simulink model "My_Model"  (R2022a)
settings: Solver=VariableStepAuto  StartTime=0.0  StopTime=10.0  RelTol=1e-3
libraries: neural x1294, spsSeriesRLCBranchLib x16, spsDiodeLib x14, spsMosfetLib x9, spsVoltageMeasurementLib x9, powerlib_extras x8, spsThreePhaseVIMeasurementLib x7, spsCurrentMeasurementLib x4, spsPVArrayLib x4, spsPWMGeneratorDCDCLib x4, spsTHDLib x4, spsThreePhaseParallelRLCBranchLib x3
(part 35 of 41)

== system My_Model/VSC Control/Current Regulator/7 layer network/Layer 3/LW{3,1} ==
  "ad{3,1}" : Inport  PortDimensions=5
      mask Display: e = 0.06;c1 = [120 230 180]/255;c2 = ([120 230 180]+0)/(256+128);c3 = ([120 230 180]+128)/(256+128);patch([0 1 1 0],[0 0 1 1],c1);patch([0 1 1 1-e 1-e 0+e],[0 0 1 1-e 0+e 0+e],c2);patch([0 0 1 1-e 0+e 0+e],[0 1 1 1-e 1-e 0+e],c3);plot([0 1 1 0 0],[0 0 1 1 0]);
  "IW{3,1}(1,:)'" : Constant  Value=[-1.8648429690334877850688144462765194475650787353515625;1.64641616981970440036775471526198089122772216796875;1.3574904436003685237466243052040226757526397705078125;0.1951467267628609059126887359525426290929317474365234375;0.67017177325838772627975004070322029292583465576171875]
      mask Display: e = 0.06;c1 = [120 150 230]/255;c2 = ([120 150 230]+0)/383;c3 = ([120 150 230]+128)/383;patch([0 1 1 0],[0 0 1 1],c1);patch([0 1 1 1-e 1-e 0+e],[0 0 1 1-e 0+e 0+e],c2);patch([0 0 1 1-e 0+e 0+e],[0 1 1 1-e 1-e 0+e],c3);plot([0 1 1 0 0],[0 0 1 1 0]);disp('weights');
  "IW{3,1}(10,:)'" : Constant  Value=[1.730384337449465181890673193265683948993682861328125;-1.493153814263745715607001329772174358367919921875;-2.530359722244460041196134625351987779140472412109375;-2.40776132219388561139794546761550009250640869140625;0.50114335757025896267435882691643200814723968505859375]
      mask Display: e = 0.06;c1 = [120 150 230]/255;c2 = ([120 150 230]+0)/383;c3 = ([120 150 230]+128)/383;patch([0 1 1 0],[0 0 1 1],c1);patch([0 1 1 1-e 1-e 0+e],[0 0 1 1-e 0+e 0+e],c2);patch([0 0 1 1-e 0+e 0+e],[0 1 1 1-e 1-e 0+e],c3);plot([0 1 1 0 0],[0 0 1 1 0]);disp('weights');
  "IW{3,1}(11,:)'" : Constant  Value=[-0.372842919851827547805811491343774832785129547119140625;-0.5046690348264208925144203021773137152194976806640625;-1.515886409077602525741212957655079662799835205078125;2.468679428778111084596957880421541631221771240234375;-1.7226432394641111311983650011825375258922576904296875]
      mask Display: e = 0.06;c1 = [120 150 230]/255;c2 = ([120 150 230]+0)/383;c3 = ([120 150 230]+128)/383;patch([0 1 1 0],[0 0 1 1],c1);patch([0 1 1 1-e 1-e 0+e],[0 0 1 1-e 0+e 0+e],c2);patch([0 0 1 1-e 0+e 0+e],[0 1 1 1-e 1-e 0+e],c3);plot([0 1 1 0 0],[0 0 1 1 0]);disp('weights');
  "IW{3,1}(12,:)'" : Constant  Value=[2.43443382104679617583542494685389101505279541015625;-2.69250576871099323028602157137356698513031005859375;-0.8594546905821596194385847411467693746089935302734375;1.642889282015585816765224080882035195827484130859375;-1.18668618700788908171261937241069972515106201171875]
      mask Display: e = 0.06;c1 = [120 150 230]/255;c2 = ([120 150 230]+0)/383;c3 = ([120 150 230]+128)/383;patch([0 1 1 0],[0 0 1 1],c1);patch([0 1 1 1-e 1-e 0+e],[0 0 1 1-e 0+e 0+e],c2);patch([0 0 1 1-e 0+e 0+e],[0 1 1 1-e 1-e 0+e],c3);plot([0 1 1 0 0],[0 0 1 1 0]);disp('weights');
  "IW{3,1}(13,:)'" : Constant  Value=[-1.866170167135730917351565949502401053905487060546875;2.372303607311231576915133700822480022907257080078125;1.88285380700856563862544135190546512603759765625;-0.057789596629258331572653872854061773978173732757568359375;-0.1485964355318751539680732776105287484824657440185546875]
      mask Display: e = 0.06;c1 = [120 150 230]/255;c2 = ([120 150 230]+0)/383;c3 = ([120 150 230]+128)/383;patch([0 1 1 0],[0 0 1 1],c1);patch([0 1 1 1-e 1-e 0+e],[0 0 1 1-e 0+e 0+e],c2);patch([0 0 1 1-e 0+e 0+e],[0 1 1 1-e 1-e 0+e],c3);plot([0 1 1 0 0],[0 0 1 1 0]);disp('weights');
  "IW{3,1}(14,:)'" : Constant  Value=[-1.22626251288648457915542167029343545436859130859375;2.309849211314865424782283298554830253124237060546875;-2.4839196222544988046365688205696642398834228515625;-0.35577383199778978006833085601101629436016082763671875;-1.38721598608713492239985498599708080291748046875]
      mask Display: e = 0.06;c1 = [120 150 230]/255;c2 = ([120 150 230]+0)/383;c3 = ([120 150 230]+128)/383;patch([0 1 1 0],[0 0 1 1],c1);patch([0 1 1 1-e 1-e 0+e],[0 0 1 1-e 0+e 0+e],c2);patch([0 0 1 1-e 0+e 0+e],[0 1 1 1-e 1-e 0+e],c3);plot([0 1 1 0 0],[0 0 1 1 0]);disp('weights');
  "IW{3,1}(15,:)'" : Constant  Value=[-2.172691293821853886214512385777197778224945068359375;-0.0555052400358548581049689119026879779994487762451171875;-2.796772108373029031014311840408481657505035400390625;-0.322606729897259025818812006036750972270965576171875;2.110627404777451143758071339107118546962738037109375]
      mask Display: e = 0.06;c1 = [120 150 230]/255;c2 = ([120 150 230]+0)/383;c3 = ([120 150 230]+128)/383;patch([0 1 1 0],[0 0 1 1],c1);patch([0 1 1 1-e 1-e 0+e],[0 0 1 1-e 0+e 0+e],c2);patch([0 0 1 1-e 0+e 0+e],[0 1 1 1-e 1-e 0+e],c3);plot([0 1 1 0 0],[0 0 1 1 0]);disp('weights');
  "IW{3,1}(16,:)'" : Constant  Value=[-1.8000723946908561146074134740047156810760498046875;-0.049744368180471336404746551806965726427733898162841796875;-1.6945002191867055696405941489501856267452239990234375;-0.93860331245166783720179637384717352688312530517578125;-1.5469042667476922137126393863582052290439605712890625]
      mask Display: e = 0.06;c1 = [120 150 230]/255;c2 = ([120 150 230]+0)/383;c3 = ([120 150 230]+128)/383;patch([0 1 1 0],[0 0 1 1],c1);patch([0 1 1 1-e 1-e 0+e],[0 0 1 1-e 0+e 0+e],c2);patch([0 0 1 1-e 0+e 0+e],[0 1 1 1-e 1-e 0+e],c3);plot([0 1 1 0 0],[0 0 1 1 0]);disp('weights');
  "IW{3,1}(17,:)'" : Constant  Value=[2.649656781046310971561297264997847378253936767578125;-1.128764384600953629700370584032498300075531005859375;0.99796670093458150763154890228179283440113067626953125;-0.014251502504089512413099072318800608627498149871826171875;-2.028262431616330463413078177836723625659942626953125]
      mask Display: e = 0.06;c1 = [120 150 230]/255;c2 = ([120 150 230]+0)/383;c3 = ([120 150 230]+128)/383;patch([0 1 1 0],[0 0 1 1],c1);patch([0 1 1 1-e 1-e 0+e],[0 0 1 1-e 0+e 0+e],c2);patch([0 0 1 1-e 0+e 0+e],[0 1 1 1-e 1-e 0+e],c3);plot([0 1 1 0 0],[0 0 1 1 0]);disp('weights');
  "IW{3,1}(18,:)'" : Constant  Value=[0.469414061379627545189663351266062818467617034912109375;2.49243645667582303104836682905443012714385986328125;1.427744966641751656055703278980217874050140380859375;0.1331815618988561322755259652694803662598133087158203125;-2.0229494597613353334963903762400150299072265625]
      mask Display: e = 0.06;c1 = [120 150 230]/255;c2 = ([120 150 230]+0)/383;c3 = ([120 150 230]+128)/383;patch([0 1 1 0],[0 0 1 1],c1);patch([0 1 1 1-e 1-e 0+e],[0 0 1 1-e 0+e 0+e],c2);patch([0 0 1 1-e 0+e 0+e],[0 1 1 1-e 1-e 0+e],c3);plot([0 1 1 0 0],[0 0 1 1 0]);disp('weights');
  "IW{3,1}(19,:)'" : Constant  Value=[0.281291509588638410921390686780796386301517486572265625;-0.73770186006364502073751054922468028962612152099609375;0.83145324988802282728528325606021098792552947998046875;1.7885333638585640958496014718548394739627838134765625;-1.539351153646769443383846009965054690837860107421875]
      mask Display: e = 0.06;c1 = [120 150 230]/255;c2 = ([120 150 230]+0)/383;c3 = ([120 150 230]+128)/383;patch([0 1 1 0],[0 0 1 1],c1);patch([0 1 1 1-e 1-e 0+e],[0 0 1 1-e 0+e 0+e],c2);patch([0 0 1 1-e 0+e 0+e],[0 1 1 1-e 1-e 0+e],c3);plot([0 1 1 0 0],[0 0 1 1 0]);disp('weights');
  "IW{3,1}(2,:)'" : Constant  Value=[2.647424845222875244843407926964573562145233154296875;0.706534071197615798354263461078517138957977294921875;-0.6292432117475985631216417459654621779918670654296875;-1.1688666566529841706056913608335889875888824462890625;-0.69896032812457409288953158466028980910778045654296875]
      mask Display: e = 0.06;c1 = [120 150 230]/255;c2 = ([120 150 230]+0)/383;c3 = ([120 150 230]+128)/383;patch([0 1 1 0],[0 0 1 1],c1);patch([0 1 1 1-e 1-e 0+e],[0 0 1 1-e 0+e 0+e],c2);patch([0 0 1 1-e 0+e 0+e],[0 1 1 1-e 1-e 0+e],c3);plot([0 1 1 0 0],[0 0 1 1 0]);disp('weights');
  "IW{3,1}(20,:)'" : Constant  Value=[-2.23870144087298594826052067219279706478118896484375;-2.4681369116425884158161352388560771942138671875;-0.327772930287947350525001866117236204445362091064453125;1.7867146454480125061792250562575645744800567626953125;-0.5014624623065147002165531375794671475887298583984375]
      mask Display: e = 0.06;c1 = [120 150 230]/255;c2 = ([120 150 230]+0)/383;c3 = ([120 150 230]+128)/383;patch([0 1 1 0],[0 0 1 1],c1);patch([0 1 1 1-e 1-e 0+e],[0 0 1 1-e 0+e 0+e],c2);patch([0 0 1 1-e 0+e 0+e],[0 1 1 1-e 1-e 0+e],c3);plot([0 1 1 0 0],[0 0 1 1 0]);disp('weights');
  "IW{3,1}(3,:)'" : Constant  Value=[-2.659172848885479112368557252921164035797119140625;-0.79211056958587333642896055607707239687442779541015625;-1.3825222862382287036808747870963998138904571533203125;1.425055984082430615700332054984755814075469970703125;1.8025932077864765812336145245353691279888153076171875]
      mask Display: e = 0.06;c1 = [120 150 230]/255;c2 = ([120 150 230]+0)/383;c3 = ([120 150 230]+128)/383;patch([0 1 1 0],[0 0 1 1],c1);patch([0 1 1 1-e 1-e 0+e],[0 0 1 1-e 0+e 0+e],c2);patch([0 0 1 1-e 0+e 0+e],[0 1 1 1-e 1-e 0+e],c3);plot([0 1 1 0 0],[0 0 1 1 0]);disp('weights');
  "IW{3,1}(4,:)'" : Constant  Value=[1.8265068772120660600677410911885090172290802001953125;0.08917576894467467429894469432838377542793750762939453125;-0.63678331617796046781876384557108394801616668701171875;-2.063555639273333408567623337148688733577728271484375;0.2208531191929975767695992772132740356028079986572265625]
      mask Display: e = 0.06;c1 = [120 150 230]/255;c2 = ([120 150 230]+0)/383;c3 = ([120 150 230]+128)/383;patch([0 1 1 0],[0 0 1 1],c1);patch([0 1 1 1-e 1-e 0+e],[0 0 1 1-e 0+e 0+e],c2);patch([0 0 1 1-e 0+e 0+e],[0 1 1 1-e 1-e 0+e],c3);plot([0 1 1 0 0],[0 0 1 1 0]);disp('weights');
  "IW{3,1}(5,:)'" : Constant  Value=[1.5732001173784180281245426158420741558074951171875;-0.43016677249347023970216241650632582604885101318359375;-2.027900356396983294615665727178566157817840576171875;1.0006433005602011210299906451837159693241119384765625;-0.72263860216961794957768461244995705783367156982421875]
      mask Display: e = 0.06;c1 = [120 150 230]/255;c2 = ([120 150 230]+0)/383;c3 = ([120 150 230]+128)/383;patch([0 1 1 0],[0 0 1 1],c1);patch([0 1 1 1-e 1-e 0+e],[0 0 1 1-e 0+e 0+e],c2);patch([0 0 1 1-e 0+e 0+e],[0 1 1 1-e 1-e 0+e],c3);plot([0 1 1 0 0],[0 0 1 1 0]);disp('weights');
  "IW{3,1}(6,:)'" : Constant  Value=[1.9049690937966279324911056392011232674121856689453125;-2.201532280789796569564487072057090699672698974609375;-1.8670742440155587704708750607096590101718902587890625;-1.56757813306267923536552189034409821033477783203125;2.4046752656764862621230349759571254253387451171875]
      mask Display: e = 0.06;c1 = [120 150 230]/255;c2 = ([120 150 230]+0)/383;c3 = ([120 150 230]+128)/383;patch([0 1 1 0],[0 0 1 1],c1);patch([0 1 1 1-e 1-e 0+e],[0 0 1 1-e 0+e 0+e],c2);patch([0 0 1 1-e 0+e 0+e],[0 1 1 1-e 1-e 0+e],c3);plot([0 1 1 0 0],[0 0 1 1 0]);disp('weights');
  "IW{3,1}(7,:)'" : Constant  Value=[-2.78018779830356610460739830159582197666168212890625;-1.8687866783189701624934286883217282593250274658203125;3.056741773225966962712618624209426343441009521484375;-0.98097265742214545536370451372931711375713348388671875;2.524511218723184402534798209671862423419952392578125]
      mask Display: e = 0.06;c1 = [120 150 230]/255;c2 = ([120 150 230]+0)/383;c3 = ([120 150 230]+128)/383;patch([0 1 1 0],[0 0 1 1],c1);patch([0 1 1 1-e 1-e 0+e],[0 0 1 1-e 0+e 0+e],c2);patch([0 0 1 1-e 0+e 0+e],[0 1 1 1-e 1-e 0+e],c3);plot([0 1 1 0 0],[0 0 1 1 0]);disp('weights');
  "IW{3,1}(8,:)'" : Constant  Value=[-0.5208757019687697553678162876167334616184234619140625;-2.0683625319881340232086586183868348598480224609375;2.446413644843494328284805305884219706058502197265625;0.6310288220066657682849609045661054551601409912109375;0.2132390764780037473169471695655374787747859954833984375]
      mask Display: e = 0.06;c1 = [120 150 230]/255;c2 = ([120 150 230]+0)/383;c3 = ([120 150 230]+128)/383;patch([0 1 1 0],[0 0 1 1],c1);patch([0 1 1 1-e 1-e 0+e],[0 0 1 1-e 0+e 0+e],c2);patch([0 0 1 1-e 0+e 0+e],[0 1 1 1-e 1-e 0+e],c3);plot([0 1 1 0 0],[0 0 1 1 0]);disp('weights');
  "IW{3,1}(9,:)'" : Constant  Value=[-1.523226272249151858062532483018003404140472412109375;-2.02999716399347374107264840858988463878631591796875;0.451636761889826210403242612301255576312541961669921875;1.8474830510928106352963595782057382166385650634765625;0.7794918762776512632939329705550335347652435302734375]
      mask Display: e = 0.06;c1 = [120 150 230]/255;c2 = ([120 150 230]+0)/383;c3 = ([120 150 230]+128)/383;patch([0 1 1 0],[0 0 1 1],c1);patch([0 1 1 1-e 1-e 0+e],[0 0 1 1-e 0+e 0+e],c2);patch([0 0 1 1-e 0+e 0+e],[0 1 1 1-e 1-e 0+e],c3);plot([0 1 1 0 0],[0 0 1 1 0]);disp('weights');
  Mux : Mux  Inputs=20
      mask Display: e = 0.06;c1 = [120 150 230]/255;c2 = ([120 150 230]+0)/383;c3 = ([120 150 230]+128)/383;patch([0 1 1 0],[0 0 1 1],c1);patch([0 1 1 1-e 1-e 0+e],[0 0 1 1-e 0+e 0+e],c2);patch([0 0 1 1-e 0+e 0+e],[0 1 1 1-e 1-e 0+e],c3);plot([0 1 1 0 0],[0 0 1 1 0]);disp('Mux');
  dotprod{1..20} (20 alike) : neural/Weight Functions/dotprod
  "lz{3,1}" : Outport
      mask Display: e = 0.06;c1 = [120 230 180]/255;c2 = ([120 230 180]+0)/(256+128);c3 = ([120 230 180]+128)/(256+128);patch([0 1 1 0],[0 0 1 1],c1);patch([0 1 1 1-e 1-e 0+e],[0 0 1 1-e 0+e 0+e],c2);patch([0 0 1 1-e 0+e 0+e],[0 1 1 1-e 1-e 0+e],c3);plot([0 1 1 0 0],[0 0 1 1 0]);
  wires:
  "IW{3,1}(1,:)'"/1 -> dotprod1/1
  "ad{3,1}"/1 -> dotprod1/2, dotprod2/2, dotprod3/2, dotprod4/2, dotprod5/2, dotprod6/2, dotprod7/2, dotprod8/2, dotprod9/2, dotprod10/2, dotprod11/2, dotprod12/2, dotprod13/2, dotprod14/2, dotprod15/2, dotprod16/2, dotprod17/2, dotprod18/2, dotprod19/2, dotprod20/2
  dotprod1/1 -> Mux/1
  "IW{3,1}(2,:)'"/1 -> dotprod2/1
  dotprod2/1 -> Mux/2
  "IW{3,1}(3,:)'"/1 -> dotprod3/1
  dotprod3/1 -> Mux/3
  "IW{3,1}(4,:)'"/1 -> dotprod4/1
  dotprod4/1 -> Mux/4
  "IW{3,1}(5,:)'"/1 -> dotprod5/1
  dotprod5/1 -> Mux/5
  "IW{3,1}(6,:)'"/1 -> dotprod6/1
  dotprod6/1 -> Mux/6
  "IW{3,1}(7,:)'"/1 -> dotprod7/1
  dotprod7/1 -> Mux/7
  "IW{3,1}(8,:)'"/1 -> dotprod8/1
  dotprod8/1 -> Mux/8
  "IW{3,1}(9,:)'"/1 -> dotprod9/1
  dotprod9/1 -> Mux/9
  "IW{3,1}(10,:)'"/1 -> dotprod10/1
  dotprod10/1 -> Mux/10
  "IW{3,1}(11,:)'"/1 -> dotprod11/1
  dotprod11/1 -> Mux/11
  "IW{3,1}(12,:)'"/1 -> dotprod12/1
  dotprod12/1 -> Mux/12
  "IW{3,1}(13,:)'"/1 -> dotprod13/1
  dotprod13/1 -> Mux/13
  "IW{3,1}(14,:)'"/1 -> dotprod14/1
  dotprod14/1 -> Mux/14
  "IW{3,1}(15,:)'"/1 -> dotprod15/1
  dotprod15/1 -> Mux/15
  "IW{3,1}(16,:)'"/1 -> dotprod16/1
  dotprod16/1 -> Mux/16
  "IW{3,1}(17,:)'"/1 -> dotprod17/1
  dotprod17/1 -> Mux/17
  "IW{3,1}(18,:)'"/1 -> dotprod18/1
  dotprod18/1 -> Mux/18
  "IW{3,1}(19,:)'"/1 -> dotprod19/1
  dotprod19/1 -> Mux/19
  "IW{3,1}(20,:)'"/1 -> dotprod20/1
  dotprod20/1 -> Mux/20
  Mux/1 -> "lz{3,1}"/1

== system My_Model/VSC Control/Current Regulator/7 layer network/Layer 3/LW{3,2} ==
  "ad{3,2}" : Inport  PortDimensions=10
      mask Display: e = 0.06;c1 = [120 230 180]/255;c2 = ([120 230 180]+0)/(256+128);c3 = ([120 230 180]+128)/(256+128);patch([0 1 1 0],[0 0 1 1],c1);patch([0 1 1 1-e 1-e 0+e],[0 0 1 1-e 0+e 0+e],c2);patch([0 0 1 1-e 0+e 0+e],[0 1 1 1-e 1-e 0+e],c3);plot([0 1 1 0 0],[0 0 1 1 0]);
  "IW{3,2}(1,:)'" : Constant  Value=[-0.9340517352811585904959201798192225396633148193359375;-1.994298770421591537882477496168576180934906005859375;-2.231733061227294978579038797761313617229461669921875;-2.2750767630508565986247049295343458652496337890625;-2.128725818503482525301251371274702250957489013671875;-1.54895013019681915267256044899113476276397705078125;2.16208710509054480297663758392445743083953857421875;-2.289238511242711826554341314476914703845977783203125;-1.2083722272665469166241791754146106541156768798828125;-0.401036443348658788732308266844484023749828338623046875]
      mask Display: e = 0.06;c1 = [120 150 230]/255;c2 = ([120 150 230]+0)/383;c3 = ([120 150 230]+128)/383;patch([0 1 1 0],[0 0 1 1],c1);patch([0 1 1 1-e 1-e 0+e],[0 0 1 1-e 0+e 0+e],c2);patch([0 0 1 1-e 0+e 0+e],[0 1 1 1-e 1-e 0+e],c3);plot([0 1 1 0 0],[0 0 1 1 0]);disp('weights');
  "IW{3,2}(10,:)'" : Constant  Value=[-0.52447000116573694317168019551900215446949005126953125;-0.2386538290880372004121312556890188716351985931396484375;1.28332790215978231884719207300804555416107177734375;0.439921775187313068844474628349416889250278472900390625;-2.013075278899036479884898653835989534854888916015625;0.74002457905065543997125132591463625431060791015625;2.776008359047869245017636785632930696010589599609375;2.0440999690321444148821683484129607677459716796875;-2.240534432538777931398499276838265359401702880859375;-1.036744034803355862806029108469374477863311767578125]
      mask Display: e = 0.06;c1 = [120 150 230]/255;c2 = ([120 150 230]+0)/383;c3 = ([120 150 230]+128)/383;patch([0 1 1 0],[0 0 1 1],c1);patch([0 1 1 1-e 1-e 0+e],[0 0 1 1-e 0+e 0+e],c2);patch([0 0 1 1-e 0+e 0+e],[0 1 1 1-e 1-e 0+e],c3);plot([0 1 1 0 0],[0 0 1 1 0]);disp('weights');
  "IW{3,2}(11,:)'" : Constant  Value=[0.53882157270662889292367481175460852682590484619140625;2.70656239894361139164402629830874502658843994140625;-2.336486569376347244286762361298315227031707763671875;-1.8986629851809009306151665441575460135936737060546875;0.94205135165820486076171391687239520251750946044921875;-1.223815999869339865568917957716621458530426025390625;-1.1431853442374391160996083272038958966732025146484375;0.80782766465166144786991253567975945770740509033203125;2.379239102210186640462552531971596181392669677734375;0.158273144072247295977007297551608644425868988037109375]
      mask Display: e = 0.06;c1 = [120 150 230]/255;c2 = ([120 150 230]+0)/383;c3 = ([120 150 230]+128)/383;patch([0 1 1 0],[0 0 1 1],c1);patch([0 1 1 1-e 1-e 0+e],[0 0 1 1-e 0+e 0+e],c2);patch([0 0 1 1-e 0+e 0+e],[0 1 1 1-e 1-e 0+e],c3);plot([0 1 1 0 0],[0 0 1 1 0]);disp('weights');
  "IW{3,2}(12,:)'" : Constant  Value=[-1.41803495722898009745449598995037376880645751953125;0.28009952932945203496473141058231703937053680419921875;0.9156131909361462373198037312249653041362762451171875;-1.55433548774674523684780069743283092975616455078125;0.09032250371490967155718720960067003034055233001708984375;-0.400164658804802952918322489495039917528629302978515625;1.196654839367555123175179687677882611751556396484375;-0.74841891289926187891268227758700959384441375732421875;2.246281987478615516096169812954030930995941162109375;0.916173888649563838981748631340451538562774658203125]
      mask Display: e = 0.06;c1 = [120 150 230]/255;c2 = ([120 150 230]+0)/383;c3 = ([120 150 230]+128)/383;patch([0 1 1 0],[0 0 1 1],c1);patch([0 1 1 1-e 1-e 0+e],[0 0 1 1-e 0+e 0+e],c2);patch([0 0 1 1-e 0+e 0+e],[0 1 1 1-e 1-e 0+e],c3);plot([0 1 1 0 0],[0 0 1 1 0]);disp('weights');
  "IW{3,2}(13,:)'" : Constant  Value=[0.62666069873449192773051663607475347816944122314453125;0.1248397322764865091659913787225377745926380157470703125;-0.017671375724152248165577105964985094033181667327880859375;2.292301081171433718708385640638880431652069091796875;2.79528636324310664207359877764247357845306396484375;-2.841105398977422868966868918505497276782989501953125;0.976535154654019521558439009822905063629150390625;-1.7912253958243715690201725010410882532596588134765625;1.8808463710691303294453291528043337166309356689453125;-0.51956649375199759344212679934571497142314910888671875]
      mask Display: e = 0.06;c1 = [120 150 230]/255;c2 = ([120 150 230]+0)/383;c3 = ([120 150 230]+128)/383;patch([0 1 1 0],[0 0 1 1],c1);patch([0 1 1 1-e 1-e 0+e],[0 0 1 1-e 0+e 0+e],c2);patch([0 0 1 1-e 0+e 0+e],[0 1 1 1-e 1-e 0+e],c3);plot([0 1 1 0 0],[0 0 1 1 0]);disp('weights');
  "IW{3,2}(14,:)'" : Constant  Value=[1.11506358881339640021224113297648727893829345703125;-1.3904828474611277133732301081181503832340240478515625;1.4270042163381957411871781005174852907657623291015625;-2.46986132485494902510936299222521483898162841796875;0.7991549146347953769264904622104950249195098876953125;2.499153695516735940174157803994603455066680908203125;0.2203053375272294445164078524612705223262310028076171875;-0.373858276178449300264361454537720419466495513916015625;-1.2230950152660542418203704073675908148288726806640625;1.6735068385839699800499147386290132999420166015625]
      mask Display: e = 0.06;c1 = [120 150 230]/255;c2 = ([120 150 230]+0)/383;c3 = ([120 150 230]+128)/383;patch([0 1 1 0],[0 0 1 1],c1);patch([0 1 1 1-e 1-e 0+e],[0 0 1 1-e 0+e 0+e],c2);patch([0 0 1 1-e 0+e 0+e],[0 1 1 1-e 1-e 0+e],c3);plot([0 1 1 0 0],[0 0 1 1 0]);disp('weights');
  "IW{3,2}(15,:)'" : Constant  Value=[-1.7074221494978922830654255449189804494380950927734375;-0.06855600666671739229496296275101485662162303924560546875;1.3116150343587573701142900972627103328704833984375;-0.06798211452282530709023689041714533232152462005615234375;1.872617615151820569252549830707721412181854248046875;-2.04539015564661763590947884949855506420135498046875;1.2256834432471432894118379408610053360462188720703125;-0.11648931484483664167139949086049455218017101287841796875;0.5729158159416700701882518842467106878757476806640625;1.3343854346625756424060682547860778868198394775390625]
      mask Display: e = 0.06;c1 = [120 150 230]/255;c2 = ([120 150 230]+0)/383;c3 = ([120 150 230]+128)/383;patch([0 1 1 0],[0 0 1 1],c1);patch([0 1 1 1-e 1-e 0+e],[0 0 1 1-e 0+e 0+e],c2);patch([0 0 1 1-e 0+e 0+e],[0 1 1 1-e 1-e 0+e],c3);plot([0 1 1 0 0],[0 0 1 1 0]);disp('weights');
  "IW{3,2}(16,:)'" : Constant  Value=[-1.9288870743812054353583107513259164988994598388671875;0.61007065719281261539919114511576481163501739501953125;2.012903545310592345884970200131647288799285888671875;-1.62491182039225545707950004725717008113861083984375;-0.281288303749119339425277530608582310378551483154296875;-1.9298024531484561094885066268034279346466064453125;0.79416010824961491554319081842550076544284820556640625;-1.8724077307737696518330494654946960508823394775390625;-2.387781861466519384151752092293463647365570068359375;2.28798201368731923821542295627295970916748046875]
      mask Display: e = 0.06;c1 = [120 150 230]/255;c2 = ([120 150 230]+0)/383;c3 = ([120 150 230]+128)/383;patch([0 1 1 0],[0 0 1 1],c1);patch([0 1 1 1-e 1-e 0+e],[0 0 1 1-e 0+e 0+e],c2);patch([0 0 1 1-e 0+e 0+e],[0 1 1 1-e 1-e 0+e],c3);plot([0 1 1 0 0],[0 0 1 1 0]);disp('weights');
  "IW{3,2}(17,:)'" : Constant  Value=[-1.513760830317681271850460689165629446506500244140625;1.2823497843177789068391803084523417055606842041015625;2.801044614029731594229133406770415604114532470703125;3.402422752220576551707154067116789519786834716796875;-0.5480754563488361430501072391052730381488800048828125;-0.959017377993459430030043222359381616115570068359375;-2.306143759193456599376759186270646750926971435546875;0.69453124753473749475318754775798879563808441162109375;-0.5192000524116686666076248002354986965656280517578125;0.1740733277058781336421589003293775022029876708984375]
      mask Display: e = 0.06;c1 = [120 150 230]/255;c2 = ([120 150 230]+0)/383;c3 = ([120 150 230]+128)/383;patch([0 1 1 0],[0 0 1 1],c1);patch([0 1 1 1-e 1-e 0+e],[0 0 1 1-e 0+e 0+e],c2);patch([0 0 1 1-e 0+e 0+e],[0 1 1 1-e 1-e 0+e],c3);plot([0 1 1 0 0],[0 0 1 1 0]);disp('weights');
  "IW{3,2}(18,:)'" : Constant  Value=[-1.1093165182660194023611666125361807644367218017578125;-0.64020626477227915440693095661117695271968841552734375;-0.99437900316058691618792408917215652763843536376953125;1.3386775871995035824824071823968552052974700927734375;2.034011846421045266453120348160155117511749267578125;-1.844827340518638170152598831919021904468536376953125;-2.29572967239675573836166222463361918926239013671875;-1.67892332731943128010243526659905910491943359375;-1.198252146307921872647739292006008327007293701171875;-1.0703407189255973452901571363327093422412872314453125]
      mask Display: e = 0.06;c1 = [120 150 230]/255;c2 = ([120 150 230]+0)/383;c3 = ([120 150 230]+128)/383;patch([0 1 1 0],[0 0 1 1],c1);patch([0 1 1 1-e 1-e 0+e],[0 0 1 1-e 0+e 0+e],c2);patch([0 0 1 1-e 0+e 0+e],[0 1 1 1-e 1-e 0+e],c3);plot([0 1 1 0 0],[0 0 1 1 0]);disp('weights');
  "IW{3,2}(19,:)'" : Constant  Value=[-0.43075615114193788190988243513857014477252960205078125;-0.7482358129670256818855023084324784576892852783203125;1.119750655590203702871576751931570470333099365234375;0.000458504026222689695969914058792937794351018965244293212890625;-2.35196176181826377415973183815367519855499267578125;-0.05938264512678835538306287844534381292760372161865234375;2.815953252733291112264168987167067825794219970703125;-0.65150215446547343756122927516116760671138763427734375;-1.910242175079114534952395842992700636386871337890625;-2.22790008566227015762706287205219268798828125]
      mask Display: e = 0.06;c1 = [120 150 230]/255;c2 = ([120 150 230]+0)/383;c3 = ([120 150 230]+128)/383;patch([0 1 1 0],[0 0 1 1],c1);patch([0 1 1 1-e 1-e 0+e],[0 0 1 1-e 0+e 0+e],c2);patch([0 0 1 1-e 0+e 0+e],[0 1 1 1-e 1-e 0+e],c3);plot([0 1 1 0 0],[0 0 1 1 0]);disp('weights');
  "IW{3,2}(2,:)'" : Constant  Value=[2.408636407640845078503843978978693485260009765625;-1.3543413755723481273207653430290520191192626953125;2.191001152204862467698376349289901554584503173828125;1.3855602038373258100278917481773532927036285400390625;1.0316818677700894113513641059398651123046875;-0.62447893619577710122570124440244399011135101318359375;2.3983715747523337569191426155157387256622314453125;0.343443140492606102665007483665249310433864593505859375;-1.1909437161203635380246623753919266164302825927734375;-2.322314414339990751301456839428283274173736572265625]
      mask Display: e = 0.06;c1 = [120 150 230]/255;c2 = ([120 150 230]+0)/383;c3 = ([120 150 230]+128)/383;patch([0 1 1 0],[0 0 1 1],c1);patch([0 1 1 1-e 1-e 0+e],[0 0 1 1-e 0+e 0+e],c2);patch([0 0 1 1-e 0+e 0+e],[0 1 1 1-e 1-e 0+e],c3);plot([0 1 1 0 0],[0 0 1 1 0]);disp('weights');
  "IW{3,2}(20,:)'" : Constant  Value=[-0.0468545440846020178060626903970842249691486358642578125;3.07045926237668265201818940113298594951629638671875;-1.9317638561219994119966258949716575443744659423828125;-0.260274585042120365496742806499241851270198822021484375;-2.3803232517256933675753316492773592472076416015625;-1.0290621511098183571419895088183693587779998779296875;-2.085445504273896855096381841576658189296722412109375;0.449346237328046793635394351440481841564178466796875;-2.05253062864685364985462001641280949115753173828125;0.60705159952966847303201802787953056395053863525390625]
      mask Display: e = 0.06;c1 = [120 150 230]/255;c2 = ([120 150 230]+0)/383;c3 = ([120 150 230]+128)/383;patch([0 1 1 0],[0 0 1 1],c1);patch([0 1 1 1-e 1-e 0+e],[0 0 1 1-e 0+e 0+e],c2);patch([0 0 1 1-e 0+e 0+e],[0 1 1 1-e 1-e 0+e],c3);plot([0 1 1 0 0],[0 0 1 1 0]);disp('weights');
  "IW{3,2}(3,:)'" : Constant  Value=[-0.289739144545416049680852665915153920650482177734375;1.64781335949918883443388040177524089813232421875;2.282609870758466552587151454645209014415740966796875;0.0815336462900848601975667406804859638214111328125;-2.413017032374254799975688001723028719425201416015625;1.842710946836365604184493349748663604259490966796875;-2.44401910281394574298019506386481225490570068359375;2.134233534409164523282242953428067266941070556640625;0.6818124364649229551815778904710896313190460205078125;0.62925223220971415738489440627745352685451507568359375]
      mask Display: e = 0.06;c1 = [120 150 230]/255;c2 = ([120 150 230]+0)/383;c3 = ([120 150 230]+128)/383;patch([0 1 1 0],[0 0 1 1],c1);patch([0 1 1 1-e 1-e 0+e],[0 0 1 1-e 0+e 0+e],c2);patch([0 0 1 1-e 0+e 0+e],[0 1 1 1-e 1-e 0+e],c3);plot([0 1 1 0 0],[0 0 1 1 0]);disp('weights');
  "IW{3,2}(4,:)'" : Constant  Value=[-2.08991144470700174196053922059945762157440185546875;-3.12565145223339868607581593096256256103515625;1.9680903228255528514267780337831936776638031005859375;-0.131811682025431198272968913443037308752536773681640625;-2.843419513005802645722042143461294472217559814453125;2.01478934226482930824886352638714015483856201171875;1.5794967306993950018068062490783631801605224609375;1.12495307516322640140060684643685817718505859375;-1.5557750427220486955093292635865509510040283203125;-0.190480433891195455320399787524365819990634918212890625]
      mask Display: e = 0.06;c1 = [120 150 230]/255;c2 = ([120 150 230]+0)/383;c3 = ([120 150 230]+128)/383;patch([0 1 1 0],[0 0 1 1],c1);patch([0 1 1 1-e 1-e 0+e],[0 0 1 1-e 0+e 0+e],c2);patch([0 0 1 1-e 0+e 0+e],[0 1 1 1-e 1-e 0+e],c3);plot([0 1 1 0 0],[0 0 1 1 0]);disp('weights');
  "IW{3,2}(5,:)'" : Constant  Value=[2.054155075119189266530383974895812571048736572265625;2.1561311280511841204088341328315436840057373046875;-1.9622354621078816894197416331735439598560333251953125;2.05586215173632869124276112415827810764312744140625;0.130717205753750287389181039543473161756992340087890625;-2.185576249373101465067747994908131659030914306640625;-1.139770102116494765454035587026737630367279052734375;-1.5065801958876845478840778014273382723331451416015625;1.6252427193852143627594841746031306684017181396484375;1.0019635344560031686711454312899149954319000244140625]
      mask Display: e = 0.06;c1 = [120 150 230]/255;c2 = ([120 150 230]+0)/383;c3 = ([120 150 230]+128)/383;patch([0 1 1 0],[0 0 1 1],c1);patch([0 1 1 1-e 1-e 0+e],[0 0 1 1-e 0+e 0+e],c2);patch([0 0 1 1-e 0+e 0+e],[0 1 1 1-e 1-e 0+e],c3);plot([0 1 1 0 0],[0 0 1 1 0]);disp('weights');
  "IW{3,2}(6,:)'" : Constant  Value=[2.618010375322563643152307122363708913326263427734375;1.217655834174616646947697518044151365756988525390625;-1.206316719712072771386601743870414793491363525390625;0.63918762392612282763337816504645161330699920654296875;-2.0126685925680565247830600128509104251861572265625;-0.5084430137299025265207319534965790808200836181640625;-0.386168516285907370555463558048359118402004241943359375;-0.64574071342870364986765707726590335369110107421875;2.540071678685621225923796373535878956317901611328125;1.142399788103536817374106249189935624599456787109375]
      mask Display: e = 0.06;c1 = [120 150 230]/255;c2 = ([120 150 230]+0)/383;c3 = ([120 150 230]+128)/383;patch([0 1 1 0],[0 0 1 1],c1);patch([0 1 1 1-e 1-e 0+e],[0 0 1 1-e 0+e 0+e],c2);patch([0 0 1 1-e 0+e 0+e],[0 1 1 1-e 1-e 0+e],c3);plot([0 1 1 0 0],[0 0 1 1 0]);disp('weights');
  "IW{3,2}(7,:)'" : Constant  Value=[-0.494041795575315745292499514107475988566875457763671875;-0.09565572377994403796552802532460191287100315093994140625;-1.2105429619885141878654621905297972261905670166015625;0.72710379851067485912352594823460094630718231201171875;2.122686587396009461059520617709495127201080322265625;0.20875082901926045320095681745442561805248260498046875;0.3306383075615120237245037060347385704517364501953125;-0.35482795744815287530826708461972884833812713623046875;1.559134186649066666774388068006373941898345947265625;0.879744916239609597852222577785141766071319580078125]
      mask Display: e = 0.06;c1 = [120 150 230]/255;c2 = ([120 150 230]+0)/383;c3 = ([120 150 230]+128)/383;patch([0 1 1 0],[0 0 1 1],c1);patch([0 1 1 1-e 1-e 0+e],[0 0 1 1-e 0+e 0+e],c2);patch([0 0 1 1-e 0+e 0+e],[0 1 1 1-e 1-e 0+e],c3);plot([0 1 1 0 0],[0 0 1 1 0]);disp('weights');
  "IW{3,2}(8,:)'" : Constant  Value=[-2.13188322626766790790497907437384128570556640625;0.40971760827243863811730761881335638463497161865234375;0.93196659887987121084762520695221610367298126220703125;1.8701144966834541971678618210717104375362396240234375;1.6472246962289152083513954494264908134937286376953125;-0.429325815202060090403080039322958327829837799072265625;2.357533413316281301064236686215735971927642822265625;2.503202446570374828382909981883130967617034912109375;-0.85785359211374656585036291289725340902805328369140625;-2.544458135388712793911736298468895256519317626953125]
      mask Display: e = 0.06;c1 = [120 150 230]/255;c2 = ([120 150 230]+0)/383;c3 = ([120 150 230]+128)/383;patch([0 1 1 0],[0 0 1 1],c1);patch([0 1 1 1-e 1-e 0+e],[0 0 1 1-e 0+e 0+e],c2);patch([0 0 1 1-e 0+e 0+e],[0 1 1 1-e 1-e 0+e],c3);plot([0 1 1 0 0],[0 0 1 1 0]);disp('weights');
  "IW{3,2}(9,:)'" : Constant  Value=[-1.5899461371197531889265519566833972930908203125;-1.7172952000737671252039717728621326386928558349609375;-2.342152045226281398271339639904908835887908935546875;1.9961918140634626883667124275234527885913848876953125;1.4597189483141927990317299190792255103588104248046875;1.0225616245271298421215533380745910108089447021484375;-0.545513716802439763142729134415276348590850830078125;-2.21927655182703720271319980383850634098052978515625;0.58868601847054058406882859344477765262126922607421875;-2.818452680638445340122189008980058133602142333984375]
      mask Display: e = 0.06;c1 = [120 150 230]/255;c2 = ([120 150 230]+0)/383;c3 = ([120 150 230]+128)/383;patch([0 1 1 0],[0 0 1 1],c1);patch([0 1 1 1-e 1-e 0+e],[0 0 1 1-e 0+e 0+e],c2);patch([0 0 1 1-e 0+e 0+e],[0 1 1 1-e 1-e 0+e],c3);plot([0 1 1 0 0],[0 0 1 1 0]);disp('weights');
  Mux : Mux  Inputs=20
      mask Display: e = 0.06;c1 = [120 150 230]/255;c2 = ([120 150 230]+0)/383;c3 = ([120 150 230]+128)/383;patch([0 1 1 0],[0 0 1 1],c1);patch([0 1 1 1-e 1-e 0+e],[0 0 1 1-e 0+e 0+e],c2);patch([0 0 1 1-e 0+e 0+e],[0 1 1 1-e 1-e 0+e],c3);plot([0 1 1 0 0],[0 0 1 1 0]);disp('Mux');
  dotprod{1..20} (20 alike) : neural/Weight Functions/dotprod
  "lz{3,2}" : Outport
      mask Display: e = 0.06;c1 = [120 230 180]/255;c2 = ([120 230 180]+0)/(256+128);c3 = ([120 230 180]+128)/(256+128);patch([0 1 1 0],[0 0 1 1],c1);patch([0 1 1 1-e 1-e 0+e],[0 0 1 1-e 0+e 0+e],c2);patch([0 0 1 1-e 0+e 0+e],[0 1 1 1-e 1-e 0+e],c3);plot([0 1 1 0 0],[0 0 1 1 0]);
  wires:
  "IW{3,2}(1,:)'"/1 -> dotprod1/1
  "ad{3,2}"/1 -> dotprod1/2, dotprod2/2, dotprod3/2, dotprod4/2, dotprod5/2, dotprod6/2, dotprod7/2, dotprod8/2, dotprod9/2, dotprod10/2, dotprod11/2, dotprod12/2, dotprod13/2, dotprod14/2, dotprod15/2, dotprod16/2, dotprod17/2, dotprod18/2, dotprod19/2, dotprod20/2
  dotprod1/1 -> Mux/1
  "IW{3,2}(2,:)'"/1 -> dotprod2/1
  dotprod2/1 -> Mux/2
  "IW{3,2}(3,:)'"/1 -> dotprod3/1
  dotprod3/1 -> Mux/3
  "IW{3,2}(4,:)'"/1 -> dotprod4/1
  dotprod4/1 -> Mux/4
  "IW{3,2}(5,:)'"/1 -> dotprod5/1
  dotprod5/1 -> Mux/5
  "IW{3,2}(6,:)'"/1 -> dotprod6/1
  dotprod6/1 -> Mux/6
  "IW{3,2}(7,:)'"/1 -> dotprod7/1
  dotprod7/1 -> Mux/7
  "IW{3,2}(8,:)'"/1 -> dotprod8/1
  dotprod8/1 -> Mux/8
  "IW{3,2}(9,:)'"/1 -> dotprod9/1
  dotprod9/1 -> Mux/9
  "IW{3,2}(10,:)'"/1 -> dotprod10/1
  dotprod10/1 -> Mux/10
  "IW{3,2}(11,:)'"/1 -> dotprod11/1
  dotprod11/1 -> Mux/11
  "IW{3,2}(12,:)'"/1 -> dotprod12/1
  dotprod12/1 -> Mux/12
  "IW{3,2}(13,:)'"/1 -> dotprod13/1
  dotprod13/1 -> Mux/13
  "IW{3,2}(14,:)'"/1 -> dotprod14/1
  dotprod14/1 -> Mux/14
  "IW{3,2}(15,:)'"/1 -> dotprod15/1
  dotprod15/1 -> Mux/15
  "IW{3,2}(16,:)'"/1 -> dotprod16/1
  dotprod16/1 -> Mux/16
  "IW{3,2}(17,:)'"/1 -> dotprod17/1
  dotprod17/1 -> Mux/17
  "IW{3,2}(18,:)'"/1 -> dotprod18/1
  dotprod18/1 -> Mux/18
  "IW{3,2}(19,:)'"/1 -> dotprod19/1
  dotprod19/1 -> Mux/19
  "IW{3,2}(20,:)'"/1 -> dotprod20/1
  dotprod20/1 -> Mux/20
  Mux/1 -> "lz{3,2}"/1

== system My_Model/VSC Control/Current Regulator/7 layer network/Layer 4/Delays 1 ==
  "p{4}" : Inport  PortDimensions=2
      mask Display: e = 0.06;c1 = [120 230 180]/255;c2 = ([120 230 180]+0)/(256+128);c3 = ([120 230 180]+128)/(256+128);patch([0 1 1 0],[0 0 1 1],c1);patch([0 1 1 1-e 1-e 0+e],[0 0 1 1-e 0+e 0+e],c2);patch([0 0 1 1-e 0+e 0+e],[0 1 1 1-e 1-e 0+e],c3);plot([0 1 1 0 0],[0 0 1 1 0]);
  mux : Mux  Inputs=1
      mask Display: e = 0.06;c1 = [120 150 230]/255;c2 = ([120 150 230]+0)/383;c3 = ([120 150 230]+128)/383;patch([0 1 1 0],[0 0 1 1],c1);patch([0 1 1 1-e 1-e 0+e],[0 0 1 1-e 0+e 0+e],c2);patch([0 0 1 1-e 0+e 0+e],[0 1 1 1-e 1-e 0+e],c3);plot([0 1 1 0 0],[0 0 1 1 0]);disp('Mux')
  "pd{4,1}" : Outport
      mask Display: e = 0.06;c1 = [120 230 180]/255;c2 = ([120 230 180]+0)/(256+128);c3 = ([120 230 180]+128)/(256+128);patch([0 1 1 0],[0 0 1 1],c1);patch([0 1 1 1-e 1-e 0+e],[0 0 1 1-e 0+e 0+e],c2);patch([0 0 1 1-e 0+e 0+e],[0 1 1 1-e 1-e 0+e],c3);plot([0 1 1 0 0],[0 0 1 1 0]);
  wires:
  "p{4}"/1 -> mux/1
  mux/1 -> "pd{4,1}"/1

== system My_Model/VSC Control/Current Regulator/7 layer network/Layer 4/Delays 2 ==
  "p{4}" : Inport  PortDimensions=5
      mask Display: e = 0.06;c1 = [120 230 180]/255;c2 = ([120 230 180]+0)/(256+128);c3 = ([120 230 180]+128)/(256+128);patch([0 1 1 0],[0 0 1 1],c1);patch([0 1 1 1-e 1-e 0+e],[0 0 1 1-e 0+e 0+e],c2);patch([0 0 1 1-e 0+e 0+e],[0 1 1 1-e 1-e 0+e],c3);plot([0 1 1 0 0],[0 0 1 1 0]);
  mux : Mux  Inputs=1
      mask Display: e = 0.06;c1 = [120 150 230]/255;c2 = ([120 150 230]+0)/383;c3 = ([120 150 230]+128)/383;patch([0 1 1 0],[0 0 1 1],c1);patch([0 1 1 1-e 1-e 0+e],[0 0 1 1-e 0+e 0+e],c2);patch([0 0 1 1-e 0+e 0+e],[0 1 1 1-e 1-e 0+e],c3);plot([0 1 1 0 0],[0 0 1 1 0]);disp('Mux')
  "pd{4,1}" : Outport
      mask Display: e = 0.06;c1 = [120 230 180]/255;c2 = ([120 230 180]+0)/(256+128);c3 = ([120 230 180]+128)/(256+128);patch([0 1 1 0],[0 0 1 1],c1);patch([0 1 1 1-e 1-e 0+e],[0 0 1 1-e 0+e 0+e],c2);patch([0 0 1 1-e 0+e 0+e],[0 1 1 1-e 1-e 0+e],c3);plot([0 1 1 0 0],[0 0 1 1 0]);
  wires:
  "p{4}"/1 -> mux/1
  mux/1 -> "pd{4,1}"/1

== system My_Model/VSC Control/Current Regulator/7 layer network/Layer 4/Delays 3 ==
  "p{4}" : Inport  PortDimensions=10
      mask Display: e = 0.06;c1 = [120 230 180]/255;c2 = ([120 230 180]+0)/(256+128);c3 = ([120 230 180]+128)/(256+128);patch([0 1 1 0],[0 0 1 1],c1);patch([0 1 1 1-e 1-e 0+e],[0 0 1 1-e 0+e 0+e],c2);patch([0 0 1 1-e 0+e 0+e],[0 1 1 1-e 1-e 0+e],c3);plot([0 1 1 0 0],[0 0 1 1 0]);
  mux : Mux  Inputs=1
      mask Display: e = 0.06;c1 = [120 150 230]/255;c2 = ([120 150 230]+0)/383;c3 = ([120 150 230]+128)/383;patch([0 1 1 0],[0 0 1 1],c1);patch([0 1 1 1-e 1-e 0+e],[0 0 1 1-e 0+e 0+e],c2);patch([0 0 1 1-e 0+e 0+e],[0 1 1 1-e 1-e 0+e],c3);plot([0 1 1 0 0],[0 0 1 1 0]);disp('Mux')
  "pd{4,2}" : Outport
      mask Display: e = 0.06;c1 = [120 230 180]/255;c2 = ([120 230 180]+0)/(256+128);c3 = ([120 230 180]+128)/(256+128);patch([0 1 1 0],[0 0 1 1],c1);patch([0 1 1 1-e 1-e 0+e],[0 0 1 1-e 0+e 0+e],c2);patch([0 0 1 1-e 0+e 0+e],[0 1 1 1-e 1-e 0+e],c3);plot([0 1 1 0 0],[0 0 1 1 0]);
  wires:
  "p{4}"/1 -> mux/1
  mux/1 -> "pd{4,2}"/1

== system My_Model/VSC Control/Current Regulator/7 layer network/Layer 4/Delays 4 ==
  "p{4}" : Inport  PortDimensions=20
      mask Display: e = 0.06;c1 = [120 230 180]/255;c2 = ([120 230 180]+0)/(256+128);c3 = ([120 230 180]+128)/(256+128);patch([0 1 1 0],[0 0 1 1],c1);patch([0 1 1 1-e 1-e 0+e],[0 0 1 1-e 0+e 0+e],c2);patch([0 0 1 1-e 0+e 0+e],[0 1 1 1-e 1-e 0+e],c3);plot([0 1 1 0 0],[0 0 1 1 0]);
  mux : Mux  Inputs=1
      mask Display: e = 0.06;c1 = [120 150 230]/255;c2 = ([120 150 230]+0)/383;c3 = ([120 150 230]+128)/383;patch([0 1 1 0],[0 0 1 1],c1);patch([0 1 1 1-e 1-e 0+e],[0 0 1 1-e 0+e 0+e],c2);patch([0 0 1 1-e 0+e 0+e],[0 1 1 1-e 1-e 0+e],c3);plot([0 1 1 0 0],[0 0 1 1 0]);disp('Mux')
  "pd{4,3}" : Outport
      mask Display: e = 0.06;c1 = [120 230 180]/255;c2 = ([120 230 180]+0)/(256+128);c3 = ([120 230 180]+128)/(256+128);patch([0 1 1 0],[0 0 1 1],c1);patch([0 1 1 1-e 1-e 0+e],[0 0 1 1-e 0+e 0+e],c2);patch([0 0 1 1-e 0+e 0+e],[0 1 1 1-e 1-e 0+e],c3);plot([0 1 1 0 0],[0 0 1 1 0]);
  wires:
  "p{4}"/1 -> mux/1
  mux/1 -> "pd{4,3}"/1
